simulink model "q1_trim"  (R2019b)
settings: Solver=VariableStepAuto  StartTime=0.0  StopTime=500.0  RelTol=1e-3
model workspace (MATLAB code in the model file):
  | q=20
  | V=1200
  | Ti=90
  | cp=0.8
  | rho=52
  | dH=-500
  | ca0=0.8
  | T0=99
settings Model: Creator=Raj  LastModifiedBy=Raj

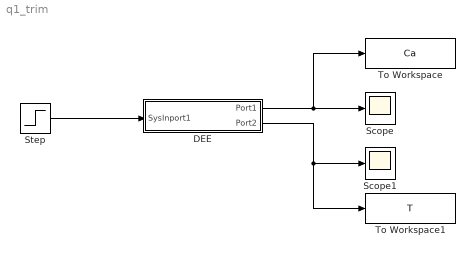
== system q1_trim ==
  DEE : Subsystem  mask(Differential Equation Editor (DEE)){}
      settings: OpenFcn=diffeqed
      mask Display: disp('CSTR')
  Scope : Scope
  Scope1 : Scope
  Step : Step  Time=5  Before=ca0  After=1.1*ca0  SampleTime=0
  To Workspace : ToWorkspace  VariableName=Ca  SaveFormat=Timeseries  SampleTime=-1
  To Workspace1 : ToWorkspace  VariableName=T  SaveFormat=Timeseries  SampleTime=-1
  wires:
  Step/1 -> DEE/1(SysInport1)
  DEE/1(Port1) -> Scope/1, To Workspace/1
  DEE/2(Port2) -> To Workspace1/1, Scope1/1

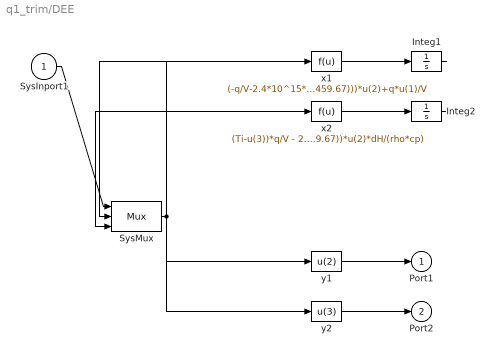
== system q1_trim/DEE ==
  SysInport1 : Inport
  Integ1 : Integrator  InitialCondition=ca0
  Integ2 : Integrator  InitialCondition=T0
  SysMux : Mux  Inputs=3
  x1 : Fcn  Expr=(-q/V-2.4*10^15*exp(-20000/(u(3)+459.67)))*u(2)+q*u(1)/V
  x2 : Fcn  Expr=(Ti-u(3))*q/V - 2.4*10^15*exp(-20000/(u(3)+459.67))*u(2)*dH/(rho*cp)
  y1 : Fcn  Expr=u(2)
  y2 : Fcn  Expr=u(3)
  Port1 : Outport
  Port2 : Outport  Port=2
  wires:
  SysInport1/1 -> SysMux/1
  SysMux/1 -> x1/1, x2/1, y1/1, y2/1
  x1/1 -> Integ1/1
  Integ1/1 -> SysMux/2
  x2/1 -> Integ2/1
  Integ2/1 -> SysMux/3
  y1/1 -> Port1/1
  y2/1 -> Port2/1
